simulink model "model_diskretizace"  (R2019b)
settings: Solver=VariableStepAuto  StartTime=0.0  StopTime=6.0  RelTol=1e-3
settings Model: Creator=Já  LastModifiedBy=Já

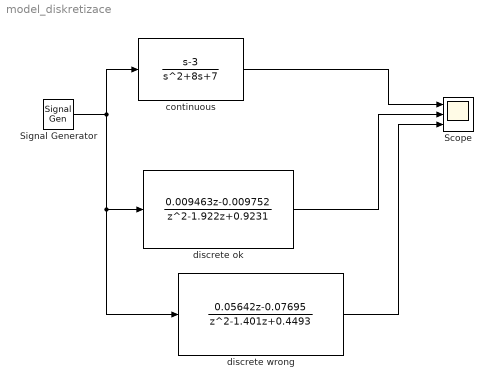
== system model_diskretizace ==
  Scope : Scope  NumInputPorts=3
  Signal Generator : SignalGenerator  WaveForm=sawtooth
  continuous : TransferFcn  Numerator=[1 -3]  Denominator=[1 8 7]
  discrete ok : DiscreteTransferFcn  Numerator=[0.009463 -0.009752]  Denominator=[1 -1.922 0.9231]  SampleTime=1/100
  discrete wrong : DiscreteTransferFcn  Numerator=[0.05642 -0.07695]  Denominator="[1  -1.401 0.4493]"  SampleTime=1/10
  wires:
  Signal Generator/1 -> discrete wrong/1, discrete ok/1, continuous/1
  discrete ok/1 -> Scope/2
  continuous/1 -> Scope/1
  discrete wrong/1 -> Scope/3
